simulink model "wheel_model_control"  (R2021a)
settings: Solver=VariableStepAuto  StartTime=0.0  StopTime=10.0  RelTol=1e-3
values from neighbouring files (symbols this model uses):
  A23 = -b*d/(a*c-b*e)    (= -1.61672463692)    [wheel_model_LQR.m]
  A43 = a*d/(a*c-b*e)    (= 39.4084774372)    [wheel_model_LQR.m]
  B21 = (c+b)/(a*c-b*e)    (= 11.3838394569)    [wheel_model_LQR.m]
  B22 = (c+b)/(a*c-b*e)    (= 11.3838394569)    [wheel_model_LQR.m]
  B41 = -(e+a)/(a*c-b*e)    (= -61.5973566863)    [wheel_model_LQR.m]
  B42 = -(e+a)/(a*c-b*e)    (= -61.5973566863)    [wheel_model_LQR.m]
  B61 = f    (= 67.610953261)    [wheel_model_LQR.m]
  B62 = -f    (= -67.610953261)    [wheel_model_LQR.m]
  K = lqr(A,B,Q,R)    [wheel_model_LQR.m]
  V = 0.5    [wheel_model_LQR.m]
  Yaw = 0    [wheel_model_LQR.m]
settings Model: Creator=solitude  LastModifiedBy=MSI_NB
settings SolverCC: AlgebraicLoopSolver=TrustRegion
settings DebuggingCC: SFMachineParentedDataDiag=warning

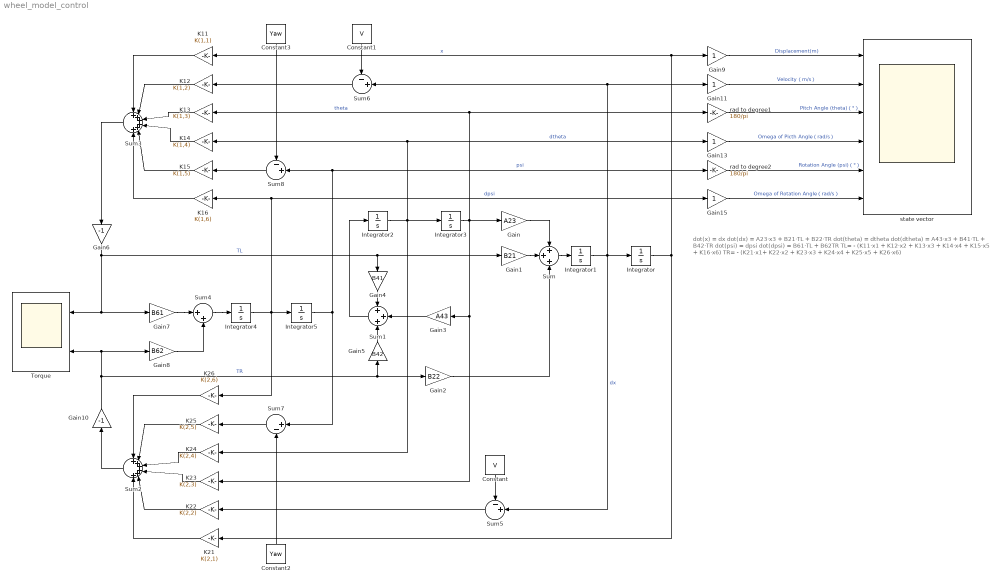
== system wheel_model_control ==
  note: dot(x) = dx
      |
      | dot(dx) = A23·x3 + B21·TL + B22·TR
      |
      | dot(theta) = dtheta
      |
      | dot(dtheta) = A43·x3 + B41·TL + B42·TR
      |
      | dot(psi) = dpsi
      |
      | dot(dpsi) = B61·TL + B62TR
      |
      | TL= - (K11·x1 + K12·x2 + K13·x3 + K14·x4 + K15·x5 + K16·x6)
      |
      | TR= - (K21·x1+ K22·x2 + K23·x3 + K24·x4 + K25·x5 + K26·x6)
  Constant : Constant  Value=V
  Constant1 : Constant  Value=V
  Constant2 : Constant  Value=Yaw
  Constant3 : Constant  Value=Yaw
  Gain : Gain  Gain=A23
  Gain1 : Gain  Gain=B21
  Gain10 : Gain  Gain=-1
  Gain{9,11,13,15} (4 alike) : Gain
  Gain2 : Gain  Gain=B22
  Gain3 : Gain  Gain=A43
  Gain4 : Gain  Gain=B41
  Gain5 : Gain  Gain=B42
  Gain6 : Gain  Gain=-1
  Gain7 : Gain  Gain=B61
  Gain8 : Gain  Gain=B62
  Integrator{,1..5} (6 alike) : Integrator
  K11 : Gain  Gain=K(1,1)
  K12 : Gain  Gain=K(1,2)
  K13 : Gain  Gain=K(1,3)
  K14 : Gain  Gain=K(1,4)
  K15 : Gain  Gain=K(1,5)
  K16 : Gain  Gain=K(1,6)
  K21 : Gain  Gain=K(2,1)
  K22 : Gain  Gain=K(2,2)
  K23 : Gain  Gain=K(2,3)
  K24 : Gain  Gain=K(2,4)
  K25 : Gain  Gain=K(2,5)
  K26 : Gain  Gain=K(2,6)
  Sum : Sum  Inputs=+++
  Sum1 : Sum  Inputs=+++
  Sum2 : Sum  Inputs=++++++
  Sum3 : Sum  Inputs=++++++
  Sum4 : Sum  Inputs=|++
  Sum5 : Sum  Inputs=-+|
  Sum6 : Sum  Inputs=-+|
  Sum7 : Sum  Inputs=|+-
  Sum8 : Sum  Inputs=-+|
  Torque : Scope  NumInputPorts=2
  rad to degree1 : Gain  Gain=180/pi
  rad to degree2 : Gain  Gain=180/pi
  state vector : Scope  NumInputPorts=6
  wires:
  Integrator/1 -> K21/1, Gain9/1, K11/1  "x"
  Integrator1/1 -> Integrator/1, Gain11/1, Sum6/2, Sum5/2  "dx"
  Integrator2/1 -> Integrator3/1, Gain13/1, K14/1, K24/1  "dtheta"
  Integrator3/1 -> Gain/1, rad to degree1/1, K13/1, Gain3/1, K23/1  "theta"
  Gain1/1 -> Sum/2
  Gain2/1 -> Sum/3
  Gain10/1 -> Torque/2, Gain8/1, Gain5/1, Gain2/1  "TR"
  Sum/1 -> Integrator1/1
  Gain4/1 -> Sum1/1
  Gain5/1 -> Sum1/3
  Sum1/1 -> Integrator2/1
  Sum2/1 -> Gain10/1
  Gain6/1 -> Gain4/1, Gain1/1, Gain7/1, Torque/1  "TL"
  K11/1 -> Sum3/1
  K12/1 -> Sum3/2
  K13/1 -> Sum3/3
  K14/1 -> Sum3/4
  Sum3/1 -> Gain6/1
  Integrator4/1 -> K16/1, Gain15/1, Integrator5/1, K26/1  "dpsi"
  Sum4/1 -> Integrator4/1
  Gain7/1 -> Sum4/1
  Gain8/1 -> Sum4/2
  Integrator5/1 -> Sum8/2, rad to degree2/1, Sum7/1  "psi"
  K15/1 -> Sum3/5
  K16/1 -> Sum3/6
  K21/1 -> Sum2/6
  K22/1 -> Sum2/5
  K23/1 -> Sum2/4
  K24/1 -> Sum2/3
  K25/1 -> Sum2/2
  K26/1 -> Sum2/1
  Sum5/1 -> K22/1
  Sum6/1 -> K12/1
  Constant1/1 -> Sum6/1
  Sum7/1 -> K25/1
  Sum8/1 -> K15/1
  Constant3/1 -> Sum8/1
  Gain9/1 -> state vector/1  "Displacement(m)"
  Gain11/1 -> state vector/2  "Velocity（m/s）"
  rad to degree1/1 -> state vector/3  "Pitch Angle (theta)（°）"
  Gain13/1 -> state vector/4  "Omega of Picth Angle（rad/s）"
  rad to degree2/1 -> state vector/5  "Rotation Angle (psi)（°）"
  Gain15/1 -> state vector/6  "Omega of Rotation Angle（rad/s）"
  Constant/1 -> Sum5/1
  Constant2/1 -> Sum7/2
  Gain3/1 -> Sum1/2
  Gain/1 -> Sum/1
